simulink model "StonkBotWithRewardModeling"  (R2021a)
settings: Solver=VariableStepAuto  StartTime=0.0  StopTime=1000  RelTol=1e-3
libraries: rllib x2
settings Model: Creator=Mitch  LastModifiedBy=Mitch

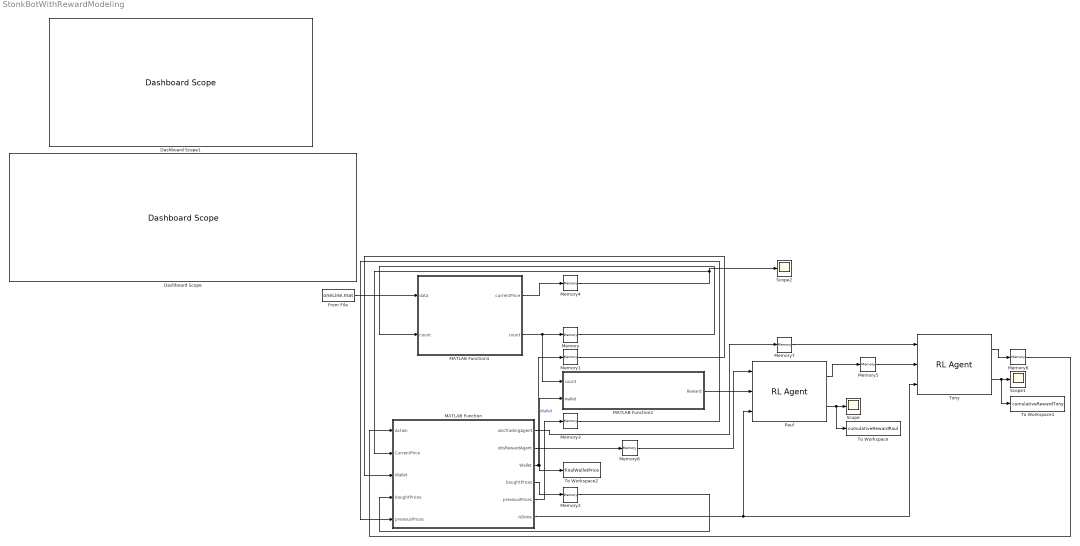
== system StonkBotWithRewardModeling ==
  Dashboard Scope : DashboardScope
  Dashboard Scope1 : DashboardScope
  From File : FromFile  FileName=oneLine.mat  SampleTime=0
  MATLAB Function : MATLAB Function  TreatAsAtomicUnit=on
  MATLAB Function1 : MATLAB Function  TreatAsAtomicUnit=on
  MATLAB Function2 : MATLAB Function  TreatAsAtomicUnit=on
  Memory : Memory  InitialCondition=1
  Memory1 : Memory  InitialCondition=500
  Memory2 : Memory  InitialCondition=[0,0,0,0,0,0,0,0]
  Memory3 : Memory  InitialCondition=[0,0,0,0,0,0,0,0]
  Memory4 : Memory
  Memory5 : Memory
  Memory6 : Memory  InitialCondition=1
  Memory7 : Memory  InitialCondition=[0,0,0,0,0,0,0,0]
  Memory8 : Memory  InitialCondition=[1,0,500]
  Paul : rllib/RL Agent  Agent=Paul  ExternalActionAsInput=off  ProvideCumRwd=on  TreatAsDirectFeedthrough=on
  Scope : Scope
  Scope1 : Scope
  Scope2 : Scope
  To Workspace : ToWorkspace  VariableName=cumulativeRewardPaul  SaveFormat=Timeseries  SampleTime=-1
  To Workspace1 : ToWorkspace  VariableName=cumulativeRewardTony  SaveFormat=Timeseries  SampleTime=-1
  To Workspace2 : ToWorkspace  VariableName=finalWalletPrice  SampleTime=-1
      settings: Save2DSignal=2-D array (concatenate along first dimension)
  Tony : rllib/RL Agent  Agent=Tony  ExternalActionAsInput=off  ProvideCumRwd=on  TreatAsDirectFeedthrough=on
  wires:
  Memory4/1 -> Scope2/1, MATLAB Function/2(CurrentPrice)
  Memory3/1 -> MATLAB Function/5("previousPrices ")
  MATLAB Function1/1(currentPrice) -> Memory4/1
  MATLAB Function/5(previousPrices) -> Memory3/1
  MATLAB Function/3(Wallet) -> MATLAB Function2/2(wallet), To Workspace2/1, Memory1/1  "Wallet"
  Memory1/1 -> MATLAB Function/3("Wallet ")
  MATLAB Function/4(boughtPrices) -> Memory2/1
  Memory2/1 -> MATLAB Function/4("boughtPrices ")
  From File/1 -> MATLAB Function1/1(data)
  Paul/1 -> Memory5/1
  Memory5/1 -> Tony/2
  MATLAB Function2/1(Reward) -> Paul/2
  Memory/1 -> MATLAB Function1/2("count ")
  Tony/1 -> Memory6/1
  Memory6/1 -> MATLAB Function/1(Action)
  MATLAB Function/1(obsTradingAgent) -> Memory7/1
  MATLAB Function/2(obsRewardAgent) -> Memory8/1
  Memory7/1 -> Tony/1
  Memory8/1 -> Paul/1
  MATLAB Function/6(isDone) -> Tony/3, Paul/3
  Paul/2 -> Scope/1, To Workspace/1
  MATLAB Function1/2(count) -> Memory/1, MATLAB Function2/1(count)
  Tony/2 -> Scope1/1, To Workspace1/1

== matlab function StonkBotWithRewardModeling/MATLAB Function1 ==
  data: data input; currentPrice output; count input; count output
function [currentPrice, count] = getDataStuff(data, count)
        
currentPrice = data(count);

count = count + 1;

end

== matlab function StonkBotWithRewardModeling/MATLAB Function ==
  data: Action input; obsTradingAgent output; CurrentPrice input; Wallet input; boughtPrices input; previousPrices input; obsRewardAgent output; Wallet output; boughtPrices output; previousPrices output; isDone output
function [obsTradingAgent, obsRewardAgent, Wallet, boughtPrices, previousPrices, isDone] = fcn(Action, CurrentPrice, Wallet, boughtPrices, previousPrices)
profit = 0;

switch(Action)
    case(1) %Buy
        Wallet = Wallet - CurrentPrice;
        boughtPrices(1:end-1) = boughtPrices(2:end);
        
        boughtPrices(end) = CurrentPrice;
        
    case(2) %Sell
        if(sum(boughtPrices) > 0)
            profit = sum(CurrentPrice - boughtPrices(boughtPrices ~= 0));
            Wallet = Wallet + profit;
            boughtPrices(:) = 0;
%             fprintf("\nCP: %3.5f | Profit: %3.5f", CurrentPrice, profit)
        end
            
    otherwise
        disp("Something is Broken: Action = " + Action)
end
    previousPrices(1:end-1) = previousPrices(2:end);

    previousPrices(end) = CurrentPrice;
    

    obsTradingAgent = [previousPrices];
    obsRewardAgent = [Action, CurrentPrice, Wallet];
    
    
    
    if(Wallet <= 0)
        isDone = 1;
    else
        isDone = 0;
    end
    
end

== matlab function StonkBotWithRewardModeling/MATLAB Function2 ==
  data: Reward output; count input; wallet input
function Reward  = trainRewardModel(count, wallet)

Reward = wallet - 500;
% if(mod(count, 10) == 0)
%  
%     
%     
% %     Reward = input("Pick a Reward amount: ");
% else
%     Reward = 0;
% end

end
